simulink subsystem "Med_PSM_Snake"  (R2023a)
settings: Solver=VariableStepAuto  StartTime=0.0  StopTime=10.0  RelTol=1e-3
model mask{baseRobot=baseRobot, q0_=q0_}
  mask prompts: q0_ "q0_ (11 dim)"
settings Model: Creator=albher  LastModifiedBy=albher

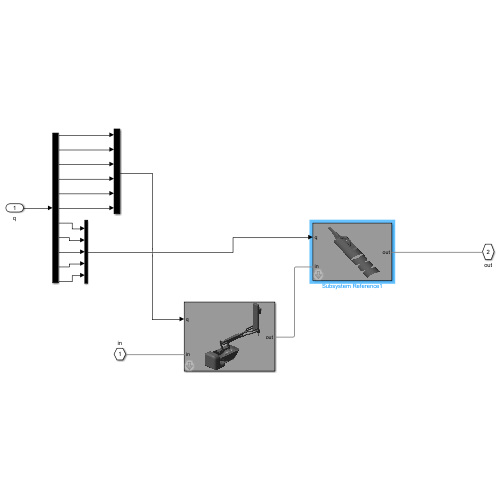
[thumbnail: Simulink's stored preview of the top-level diagram]
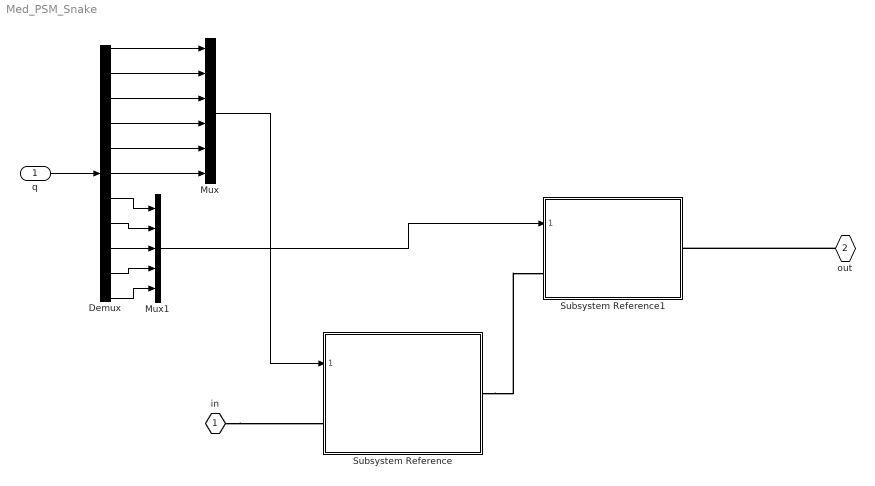
== system Med_PSM_Snake ==
  q : Inport
  Demux : Demux  Outputs=11
  Mux : Mux  Inputs=6
  Mux1 : Mux  Inputs=5
  Subsystem Reference : Subsystem  ReferencedSubsystem=Med_PSM  baseRobot=baseRobot  q0_=q0_(1:6)
  Subsystem Reference1 : Subsystem  ReferencedSubsystem=Med_Snake  baseRobot=zeros(1,6)  q0_=q0_(7:11)
  in : PMIOPort  Side=Left
  out : PMIOPort  Port=2  Side=Right
  wires:
  Demux/1 -> Mux/1
  Demux/2 -> Mux/2
  Demux/3 -> Mux/3
  Demux/4 -> Mux/4
  Demux/5 -> Mux/5
  Demux/6 -> Mux/6
  Demux/7 -> Mux1/1
  Demux/8 -> Mux1/2
  Demux/9 -> Mux1/3
  Demux/10 -> Mux1/4
  Demux/11 -> Mux1/5
  q/1 -> Demux/1
  Mux1/1 -> Subsystem Reference1/1
  Mux/1 -> Subsystem Reference/1
  connections:
  out/RConn1 -- Subsystem Reference1/RConn1
  in/RConn1 -- Subsystem Reference/LConn1
  Subsystem Reference/RConn1 -- Subsystem Reference1/LConn1
